simulink model "pcssp_KCURR_PFPO1_for_MUSCLE3"  (R2023b)
settings: configuration reference "configurationSettings" (kept outside this file)
undefined symbols (not defined in the file or in its folder): DiscIntNeverNeededParam, KCURR_PFPO1_fp, KCURR_PFPO1_tp, ParameterScheduling_KCURR, PCSSP_KCURR_ext_sizes
libraries: simulink x4
(part 2 of 2)

== matlab function pcssp_KCURR_PFPO1_for_MUSCLE3/ParameterSchedulingRegion ==
  data: p input size=1; Region output; ParameterScheduling_KCURR parameter; PCSSP_KCURR_ext_sizes parameter
function Region = ParamThr4Scheduling(p,ParameterScheduling_KCURR,PCSSP_KCURR_ext_sizes)
%#codegen

Np = PCSSP_KCURR_ext_sizes.scheduling_var;
persistent isinbandold levelold

% clear/init persistent variables
if isempty(isinbandold)
    isinbandold = NaN*ones(Np,1);
    levelold = NaN*ones(Np,1);
end

% pre-allocate sizes
isinterval = zeros(Np,1);
intervalLB =  zeros(Np,1);
intervalUB = zeros(Np,1);
isinLB = zeros(Np,1);
isinUB =  zeros(Np,1);
isinband =  zeros(Np,1);
activeband = ones(Np,1)*[-1e10 -1e9];
level = NaN*ones(Np,1);
for k = 1:Np
    if p(k) > ParameterScheduling_KCURR(k).max
        p(k) = ParameterScheduling_KCURR(k).max;
    elseif p(k) < ParameterScheduling_KCURR(k).min
        p(k) = ParameterScheduling_KCURR(k).min;
    end

    isinterval(k) = find(p(k) >= ParameterScheduling_KCURR(k).levels(1:ParameterScheduling_KCURR.Nlevels-1) && p(k)<= ParameterScheduling_KCURR(k).levels(2:ParameterScheduling_KCURR.Nlevels),1);

    if isnan(levelold(k))
        levelold(k) = isinterval(k);
    end
    if ParameterScheduling_KCURR(k).isHysteresis
        intervalLB(k) = ParameterScheduling_KCURR(k).levels(isinterval(k));
        intervalUB(k) = ParameterScheduling_KCURR(k).levels(isinterval(k)+1);
        isinLB(k) = p(k)<=intervalLB(k)+ParameterScheduling_KCURR(k).HysteresisDeltaBoundary;
        isinUB(k) = p(k)>=intervalUB(k)-ParameterScheduling_KCURR(k).HysteresisDeltaBoundary;
        if isinLB(k)
            isinband(k) = 1;
        elseif isinUB(k)
            isinband(k) = 1;
        else
            isinband(k) = 0;
        end
        
        if isempty(isinbandold(k))
            isinbandold(k) = isinband(k);
        end
        if isinbandold(k) == isinband(k)
            level(k) = levelold(k);
        else
            level(k) = isinterval(k);
        end
        levelold(k) = level(k);
        isinbandold(k) = isinband(k);
    else
        level(k) = isinterval(k);
    end
end
Region = level;
